simulink model "problem1"  (R2020b)
settings: Solver=VariableStepAuto  StartTime=0.0  StopTime=10.0  RelTol=1e-3
settings Model: Creator=Akshata Ashok  LastModifiedBy=Akshata Ashok

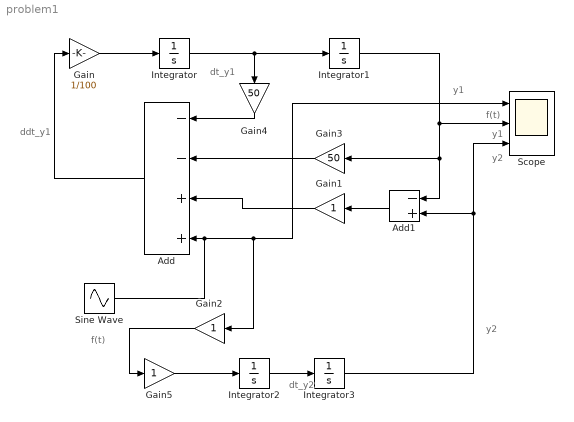
== system problem1 ==
  note: y2
  note: dt_y2
  note: y1
  note: y2
  note: f(t)
  note: y1
  note: f(t)
  note: ddt_y1
  note: dt_y1
  Add : Sum  Inputs=--++
  Add1 : Sum  Inputs=-+
  Gain : Gain  Gain=1/100
  Gain1 : Gain
  Gain2 : Gain
  Gain3 : Gain  Gain=50
  Gain4 : Gain  Gain=50
  Gain5 : Gain
  Integrator{,1..3} (4 alike) : Integrator
  Scope : Scope  NumInputPorts=3
  Sine Wave : Sin  Amplitude=2  Frequency=10  SampleTime=0
  wires:
  Integrator/1 -> Gain4/1, Integrator1/1
  Gain/1 -> Integrator/1
  Gain4/1 -> Add/1
  Gain3/1 -> Add/2
  Gain1/1 -> Add/3
  Sine Wave/1 -> Gain2/1, Scope/1, Add/4
  Gain2/1 -> Gain5/1
  Gain5/1 -> Integrator2/1
  Integrator2/1 -> Integrator3/1
  Add1/1 -> Gain1/1
  Integrator3/1 -> Add1/2, Scope/3
  Integrator1/1 -> Gain3/1, Add1/1, Scope/2
  Add/1 -> Gain/1
